simulink subsystem "rangeCheck"  (R2022a)
settings: Solver=VariableStepAuto  StartTime=0.0  StopTime=10.0  RelTol=1e-3
settings Model: Creator=janbantle  LastModifiedBy=janbantle

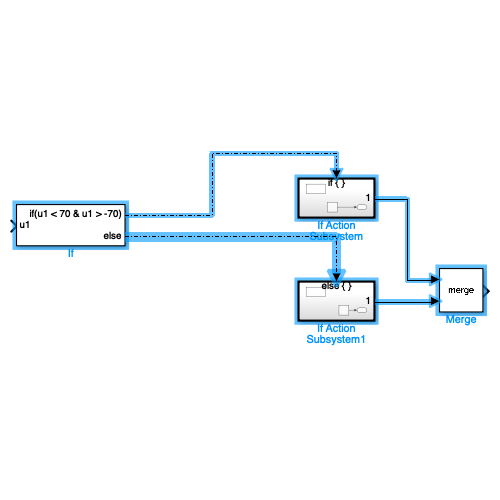
[thumbnail: Simulink's stored preview of the top-level diagram]
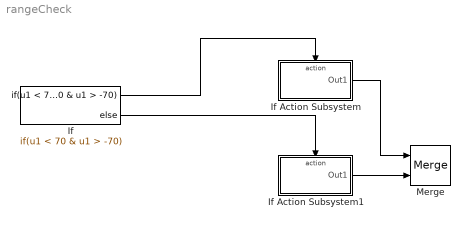
== system rangeCheck ==
  If : If  IfExpression=u1 < 70 & u1 > -70
  If Action Subsystem : Subsystem  TreatAsAtomicUnit=on
  If Action Subsystem1 : Subsystem  TreatAsAtomicUnit=on
  Merge : Merge
  wires:
  If Action Subsystem1/1(Out1) -> Merge/2
  If/1 -> If Action Subsystem/Action
  If Action Subsystem/1(Out1) -> Merge/1
  If/2 -> If Action Subsystem1/Action

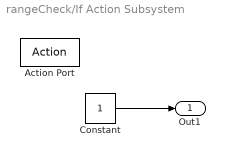
== system rangeCheck/If Action Subsystem ==
  Action Port : ActionPort  ActionPortLabel=if(u1 < 70 & u1 > -70)
  Constant : Constant
  Out1 : Outport
  wires:
  Constant/1 -> Out1/1

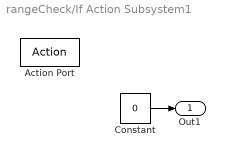
== system rangeCheck/If Action Subsystem1 ==
  Action Port : ActionPort  ActionPortLabel=else
  Constant : Constant  Value=0
  Out1 : Outport
  wires:
  Constant/1 -> Out1/1
